simulink model "pjh_pid"  (R2020a)
settings: Solver=FixedStepAuto  StartTime=0.0  StopTime=inf  FixedStep=SAMPLE_TIME  RelTol=1e-3
undefined symbols (not defined in the file or in its folder): D_saturation, DiscIntNeverNeededParam, G_correct_gain, GEAR_RATIO, I_saturation, Kpid, Ktaud, MAX_QD, MAX_QDD, MAX_TAU, MJ_Test1_torque_mode, N, N_PLoop, N_VLoop, NUM_SEGMS, P_Kp, P_saturation, q_zero_offset, SAMPLE_TIME, theta_max, theta_min, v_des_saturation, V_Kd, V_Ki, V_Kp, v_threshold_I_stop
libraries: ighEthercatLib x38, simulink x7, simulink_extras x5, dspstat3 x3
(part 2 of 2)

== system pjh_pid/Enabled Subsystem1 ==
  In1 : Inport
  Enable : EnablePort
  Out1 : Outport
  wires:
  In1/1 -> Out1/1

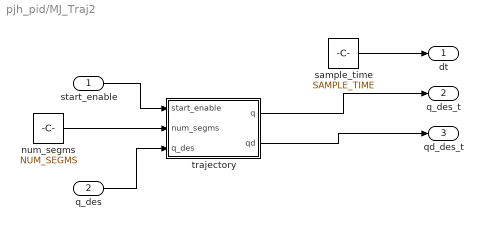
== system pjh_pid/MJ_Traj2 ==
  start_enable : Inport
  q_des : Inport  Port=2
  num_segms : Constant  Value=NUM_SEGMS
  sample_time : Constant  Value=SAMPLE_TIME
  trajectory : Subsystem
  dt : Outport
  q_des_t : Outport  Port=2
  qd_des_t : Outport  Port=3
  wires:
  sample_time/1 -> dt/1
  trajectory/1(q) -> q_des_t/1
  trajectory/2(qd) -> qd_des_t/1
  num_segms/1 -> trajectory/2(num_segms)
  start_enable/1 -> trajectory/1(start_enable)
  q_des/1 -> trajectory/3(q_des)

== system pjh_pid/Model Source ==

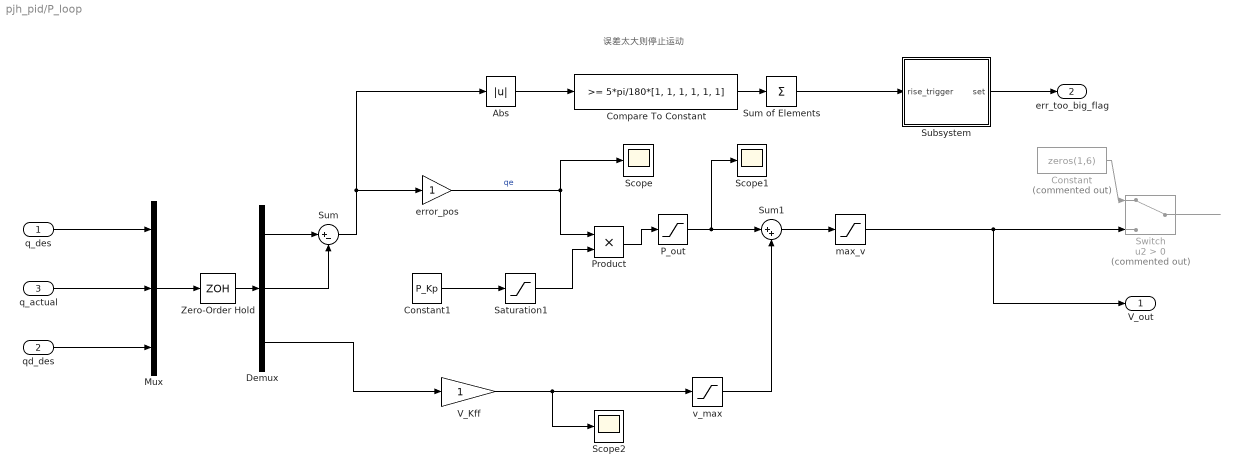
== system pjh_pid/P_loop ==
  note: 误差太大则停止运动
  q_des : Inport
  qd_des : Inport  Port=2
  q_actual : Inport  Port=3
  Abs : Abs
  Compare To Constant : simulink/Logic and Bit Operations/Compare To Constant  relop=>=  const=5*pi/180*[1, 1, 1, 1, 1, 1]  OutDataTypeStr=boolean
  Constant : Constant  Commented=on  Value=zeros(1,6)
  Constant1 : Constant  Value=P_Kp
  Demux : Demux  Outputs=[6 6 6]
  Mux : Mux  Inputs=3
  P_out : Saturate  UpperLimit=MAX_QD*0.8  LowerLimit=-MAX_QD*0.8
  Product : Product
  Saturation1 : Saturate  UpperLimit=50*ones(1,6)  LowerLimit=zeros(1,6)
  Scope : Scope
  Scope1 : Scope
  Scope2 : Scope
  Subsystem : Subsystem
  Sum : Sum  Inputs=|+-
  Sum of Elements : Sum  Inputs=+
  Sum1 : Sum  Inputs=|++
  Switch : Switch  Commented=on  Criteria=u2 > Threshold
  V_Kff : Gain
  Zero-Order Hold : ZeroOrderHold  SampleTime=SAMPLE_TIME*N_PLoop
  error_pos : Gain
  max_v : Saturate  UpperLimit=MAX_QD*4  LowerLimit=-MAX_QD*4
  v_max : Saturate  UpperLimit=MAX_QD*2  LowerLimit=-MAX_QD*2
  V_out : Outport
  err_too_big_flag : Outport  Port=2
  wires:
  Demux/1 -> Sum/1
  Product/1 -> P_out/1
  Demux/2 -> Sum/2
  Demux/3 -> V_Kff/1
  V_Kff/1 -> Scope2/1, v_max/1
  Sum1/1 -> max_v/1
  q_des/1 -> Mux/1
  q_actual/1 -> Mux/2
  qd_des/1 -> Mux/3
  Mux/1 -> Zero-Order Hold/1
  Zero-Order Hold/1 -> Demux/1
  max_v/1 -> V_out/1, Switch/3
  error_pos/1 -> Product/1, Scope/1  "qe"
  P_out/1 -> Sum1/1, Scope1/1
  Sum/1 -> error_pos/1, Abs/1
  v_max/1 -> Sum1/2
  Abs/1 -> Compare To Constant/1
  Switch/1 -> ?
  Constant/1 -> Switch/1
  Sum of Elements/1 -> Subsystem/1(rise_trigger)
  Compare To Constant/1 -> Sum of Elements/1
  Subsystem/1(set) -> err_too_big_flag/1
  Constant1/1 -> Saturation1/1
  Saturation1/1 -> Product/2

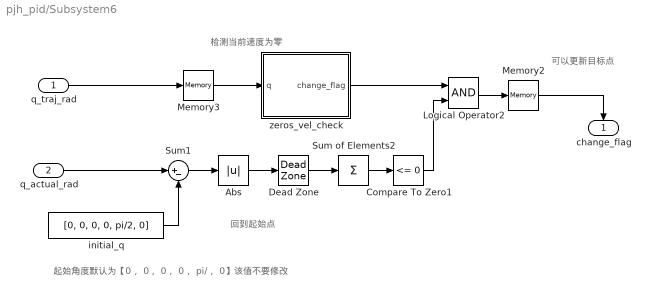
== system pjh_pid/Subsystem6 ==
  note: 起始角度默认为【0， 0， 0， 0， pi/， 0】该值不要修改
  note: 可以更新目标点
  note: 回到起始点
  note: 检测当前速度为零
  q_traj_rad : Inport
  q_actual_rad : Inport  Port=2
  Abs : Abs
  Compare To Zero1 : simulink/Logic and Bit Operations/Compare To Zero  relop=<=  OutDataTypeStr=boolean
  Dead Zone : DeadZone  LowerValue=zeros(1,6)  UpperValue=2*pi/180*[1, 1, 1, 1, 1, 1]  SaturateOnIntegerOverflow=on
  Logical Operator2 : Logic  AllPortsSameDT=off  OutDataTypeStr=boolean
  Memory2 : Memory  InitialCondition=1  InheritSampleTime=on
  Memory3 : Memory  InitialCondition=[0, 0, 0, 0, pi/2, 0]  InheritSampleTime=on
  Sum of Elements2 : Sum  Inputs=+
  Sum1 : Sum  Inputs=|+-
  initial_q : Constant  Value=[0, 0, 0, 0, pi/2, 0]
  zeros_vel_check : Subsystem
  change_flag : Outport
  wires:
  Logical Operator2/1 -> Memory2/1
  q_actual_rad/1 -> Sum1/1
  Abs/1 -> Dead Zone/1
  initial_q/1 -> Sum1/2
  Sum of Elements2/1 -> Compare To Zero1/1
  Compare To Zero1/1 -> Logical Operator2/2
  Sum1/1 -> Abs/1
  Dead Zone/1 -> Sum of Elements2/1
  zeros_vel_check/1(change_flag) -> Logical Operator2/1
  Memory3/1 -> zeros_vel_check/1(q)
  Memory2/1 -> change_flag/1
  q_traj_rad/1 -> Memory3/1

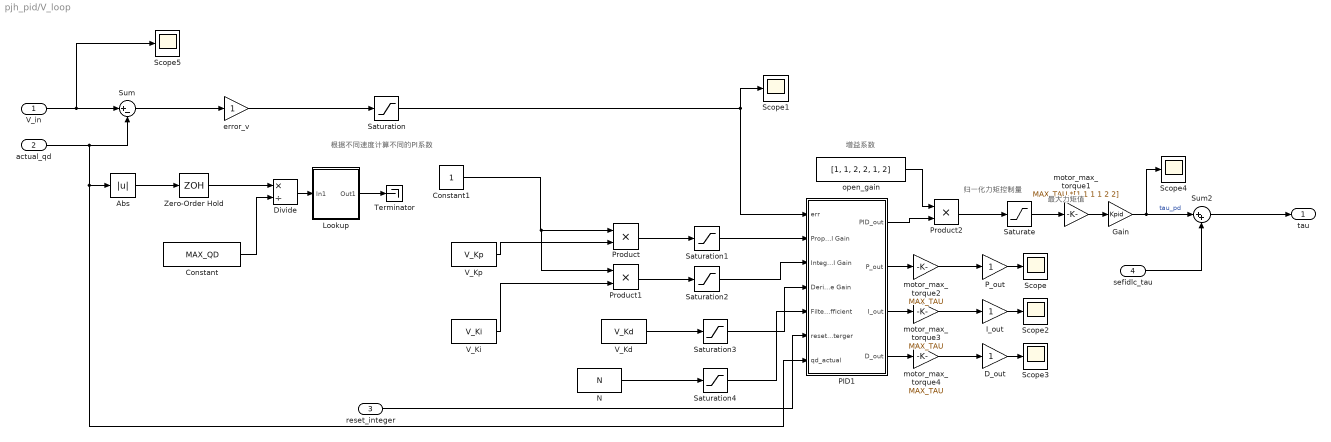
== system pjh_pid/V_loop ==
  note: 归一化力矩控制量
  note: 最大力矩值
  note: 增益系数
  note: 根据不同速度计算不同的PI系数
  V_in : Inport
  actual_qd : Inport  Port=2
  reset_integer : Inport  Port=3
  sefidlc_tau : Inport  Port=4
  " Lookup" : Subsystem
  Abs : Abs
  Constant : Constant  Value=MAX_QD
  Constant1 : Constant
  D_out : Gain
  Divide : Product  Inputs=*/
  Gain : Gain  Gain=Kpid
  I_out : Gain
  N : Constant  Value=N
  PID1 : Subsystem  AncestorBlock=simulink/Continuous/PID Controller  DialogController=pidpack.PIDConfig.pidDDGCreate
      settings: DeleteFcn=pidpack.PIDConfig.closeTuner(gcbh)  ModelCloseFcn=pidpack.PIDConfig.closeTuner(gcbh)  NameChangeFcn=pidpack.PIDConfig.updateTunerName(gcbh)
  P_out : Gain
  Product : Product
  Product1 : Product
  Product2 : Product
  Saturate : Saturate  UpperLimit=ones(1,6)  LowerLimit=-ones(1,6)
  Saturation : Saturate  UpperLimit=v_des_saturation*4  LowerLimit=-v_des_saturation*4
  Saturation1 : Saturate  UpperLimit=[10, 10, 10, 10, 10, 10]  LowerLimit=[0, 0, 0, 0, 0, 0]
  Saturation2 : Saturate  UpperLimit=200*[1, 1, 1, 1, 1, 1]  LowerLimit=[0, 0, 0, 0, 0, 0]
  Saturation3 : Saturate  UpperLimit=[10, 10, 10, 10, 10, 10]  LowerLimit=[0, 0, 0, 0, 0, 0]
  Saturation4 : Saturate  UpperLimit=[10, 10, 10, 10, 10, 10]  LowerLimit=[0, 0, 0, 0, 0, 0]
  Scope{,1..5} (6 alike) : Scope
  Sum : Sum  Inputs=|+-
  Sum2 : Sum  Inputs=|++
  Terminator : Terminator
  V_Kd : Constant  Value=V_Kd
  V_Ki : Constant  Value=V_Ki
  V_Kp : Constant  Value=V_Kp
  Zero-Order Hold : ZeroOrderHold  SampleTime=SAMPLE_TIME
  error_v : Gain
  motor_max_torque1 : Gain  Gain=MAX_TAU.*[1 1 1 1 2 2]
  motor_max_torque2 : Gain  Gain=MAX_TAU
  motor_max_torque3 : Gain  Gain=MAX_TAU
  motor_max_torque4 : Gain  Gain=MAX_TAU
  open_gain : Constant  Value=[1, 1, 2, 2, 1, 2]
  tau : Outport
  wires:
  V_in/1 -> Sum/1, Scope5/1
  actual_qd/1 -> PID1/7(qd_actual), Abs/1, Sum/2
  motor_max_torque1/1 -> Gain/1
  Sum/1 -> error_v/1
  error_v/1 -> Saturation/1
  Saturation/1 -> PID1/1(err), Scope1/1
  Saturation1/1 -> PID1/2(Proportional Gain)
  V_Kd/1 -> Saturation3/1
  N/1 -> Saturation4/1
  PID1/2(P_out) -> motor_max_torque2/1
  PID1/3(I_out) -> motor_max_torque3/1
  PID1/4(D_out) -> motor_max_torque4/1
  Product2/1 -> Saturate/1
  Product/1 -> Saturation1/1
  Saturation2/1 -> PID1/3(Integral Gain)
  Saturation3/1 -> PID1/4(Derivative Gain)
  Saturation4/1 -> PID1/5(Filter Coefficient)
  Abs/1 -> Zero-Order Hold/1
  Constant/1 -> Divide/2
  Divide/1 -> " Lookup"/1(In1)
  Zero-Order Hold/1 -> Divide/1
  motor_max_torque2/1 -> P_out/1
  Product1/1 -> Saturation2/1
  open_gain/1 -> Product2/1
  reset_integer/1 -> PID1/6(reset_interger)
  Sum2/1 -> tau/1
  V_Kp/1 -> Product/2
  V_Ki/1 -> Product1/2
  PID1/1(PID_out) -> Product2/2
  Saturate/1 -> motor_max_torque1/1
  Constant1/1 -> Product1/1, Product/1
  " Lookup"/1(Out1) -> Terminator/1
  P_out/1 -> Scope/1
  I_out/1 -> Scope2/1
  motor_max_torque3/1 -> I_out/1
  D_out/1 -> Scope3/1
  motor_max_torque4/1 -> D_out/1
  Gain/1 -> Scope4/1, Sum2/1  "tau_pd"
  sefidlc_tau/1 -> Sum2/2

== system pjh_pid/inc2rad ==
  inc : Inport
  Constant : Constant
  Divide : Product  Inputs=*/
  gear_ratio : Gain  Gain=GEAR_RATIO
  rad2inc : Gain  Gain=2^17/(2*pi)
  rad : Outport
  wires:
  gear_ratio/1 -> rad2inc/1
  rad2inc/1 -> Divide/2
  Constant/1 -> gear_ratio/1
  Divide/1 -> rad/1
  inc/1 -> Divide/1

== system pjh_pid/inc2rad1 ==
  inc : Inport
  Constant : Constant
  Divide : Product  Inputs=*/
  gear_ratio : Gain  Gain=GEAR_RATIO
  rad2inc : Gain  Gain=2^17/(2*pi)
  rad : Outport
  wires:
  inc/1 -> Divide/1
  Divide/1 -> rad/1
  Constant/1 -> gear_ratio/1
  rad2inc/1 -> Divide/2
  gear_ratio/1 -> rad2inc/1

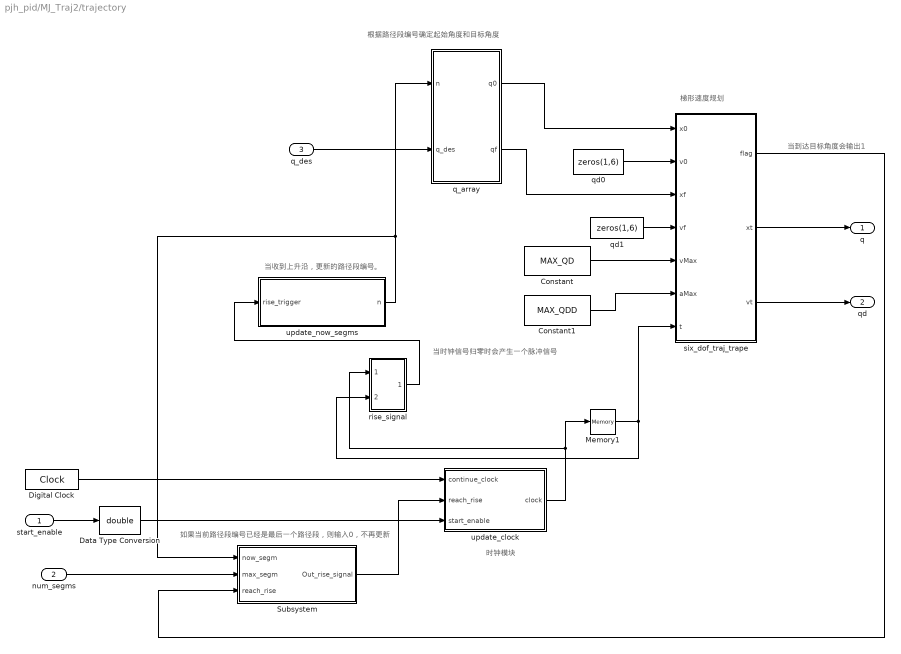
== system pjh_pid/MJ_Traj2/trajectory ==
  note: 如果当前路径段编号已经是最后一个路径段，则输入0，不再更新
  note: 当到达目标角度会输出1
  note: 根据路径段编号确定起始角度和目标角度
  note: 当收到上升沿，更新的路径段编号。
  note: 当时钟信号归零时会产生一个脉冲信号
  note: 时钟模块
  note: 梯形速度规划
  start_enable : Inport
  num_segms : Inport  Port=2
  q_des : Inport  Port=3
  Constant : Constant  Value=MAX_QD
  Constant1 : Constant  Value=MAX_QDD
  Data Type Conversion : DataTypeConversion  OutDataTypeStr=double
  Digital Clock : DigitalClock  SampleTime=SAMPLE_TIME
  Memory1 : Memory
  Subsystem : Subsystem
  q_array : MATLAB Function  TreatAsAtomicUnit=on  SystemSampleTime=SAMPLE_TIME
  qd0 : Constant  Value=zeros(1,6)
  qd1 : Constant  Value=zeros(1,6)
  rise_signal : Subsystem
  six_dof_traj_trape : MATLAB Function  TreatAsAtomicUnit=on
  update_clock : Subsystem
  update_now_segms : Subsystem
  q : Outport
  qd : Outport  Port=2
  wires:
  q_array/2(qf) -> six_dof_traj_trape/3(xf)
  Digital Clock/1 -> update_clock/1(continue_clock)
  Memory1/1 -> six_dof_traj_trape/7(t), rise_signal/2(In2)
  q_array/1(q0) -> six_dof_traj_trape/1(x0)
  rise_signal/1(Out1) -> update_now_segms/1(rise_trigger)
  update_clock/1(clock) -> rise_signal/1(In1), Memory1/1
  Subsystem/1(Out_rise_signal) -> update_clock/2(reach_rise)
  num_segms/1 -> Subsystem/2(max_segm)
  update_now_segms/1(n) -> q_array/1(n), Subsystem/1(now_segm)
  six_dof_traj_trape/2(xt) -> q/1
  six_dof_traj_trape/3(vt) -> qd/1
  qd0/1 -> six_dof_traj_trape/2(v0)
  qd1/1 -> six_dof_traj_trape/4(vf)
  six_dof_traj_trape/1(flag) -> Subsystem/3(reach_rise)
  Data Type Conversion/1 -> update_clock/3(start_enable)
  start_enable/1 -> Data Type Conversion/1
  q_des/1 -> q_array/2(q_des)
  Constant/1 -> six_dof_traj_trape/5(vMax)
  Constant1/1 -> six_dof_traj_trape/6(aMax)

== system pjh_pid/P_loop/Subsystem ==
  rise_trigger : Inport
  Constant1 : Constant
  Memory2 : Memory  InheritSampleTime=on
  Triggered Subsystem1 : Subsystem  TreatAsAtomicUnit=on
  set : Outport
  wires:
  rise_trigger/1 -> Triggered Subsystem1/Trigger
  Triggered Subsystem1/1(Out1) -> Memory2/1
  Constant1/1 -> Triggered Subsystem1/1(In1)
  Memory2/1 -> set/1

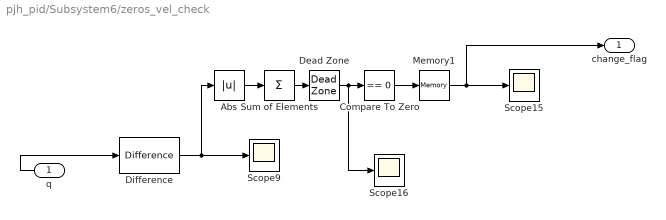
== system pjh_pid/Subsystem6/zeros_vel_check ==
  q : Inport
  Abs : Abs
  Compare To Zero : simulink/Logic and Bit Operations/Compare To Zero  relop===  OutDataTypeStr=boolean
  Dead Zone : DeadZone  LowerValue=0  UpperValue=0.0001  SaturateOnIntegerOverflow=on
  Difference : simulink/Discrete/Difference  ICPrevInput=zeros(1,6)  OutMin=[]  OutMax=[]  OutDataType=fixdt(1, 16)  OutScaling=2^-10  DoSatur=off
  Memory1 : Memory  InitialCondition=1  InheritSampleTime=on
  Scope15 : Scope
  Scope16 : Scope
  Scope9 : Scope
  Sum of Elements : Sum  Inputs=+
  change_flag : Outport
  wires:
  q/1 -> Difference/1
  Abs/1 -> Sum of Elements/1
  Dead Zone/1 -> Compare To Zero/1, Scope16/1
  Memory1/1 -> change_flag/1, Scope15/1
  Difference/1 -> Scope9/1, Abs/1
  Compare To Zero/1 -> Memory1/1
  Sum of Elements/1 -> Dead Zone/1

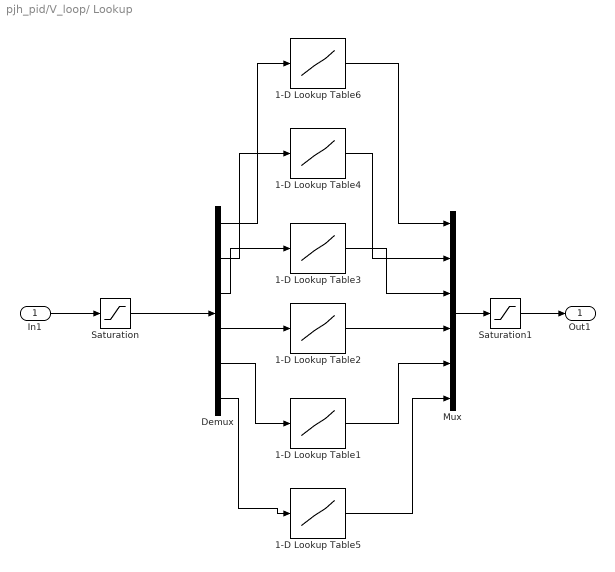
== system pjh_pid/V_loop/ Lookup ==
  In1 : Inport
  1-D Lookup Table{1..4,6} (5 alike) : Lookup_n-D  NumberOfTableDimensions=1  BreakpointsForDimension1=[0, 0.1,0.2, 0.3, 0.4, 1 ]  Table=[1, 1, 0.8, 0.6, 0.5, 0.5]  InternalRulePriority=Speed  RndMeth=Simplest  InputSameDT=on
  1-D Lookup Table5 : Lookup_n-D  NumberOfTableDimensions=1  BreakpointsForDimension1=[0, 0.1,0.2, 0.3, 0.4, 1 ]  Table=[1, 1, 1, 1, 1, 1]  InternalRulePriority=Speed  RndMeth=Simplest  InputSameDT=on
  Demux : Demux  Outputs=6
  Mux : Mux  Inputs=6
  Saturation : Saturate  UpperLimit=ones(1,6)  LowerLimit=zeros(1,6)
  Saturation1 : Saturate  UpperLimit=5*ones(1,6)  LowerLimit=zeros(1,6)
  Out1 : Outport
  wires:
  1-D Lookup Table6/1 -> Mux/1
  Demux/1 -> 1-D Lookup Table6/1
  In1/1 -> Saturation/1
  Demux/2 -> 1-D Lookup Table4/1
  Demux/3 -> 1-D Lookup Table3/1
  Demux/4 -> 1-D Lookup Table2/1
  Demux/5 -> 1-D Lookup Table1/1
  Demux/6 -> 1-D Lookup Table5/1
  Saturation/1 -> Demux/1
  1-D Lookup Table4/1 -> Mux/2
  1-D Lookup Table3/1 -> Mux/3
  1-D Lookup Table2/1 -> Mux/4
  1-D Lookup Table1/1 -> Mux/5
  1-D Lookup Table5/1 -> Mux/6
  Saturation1/1 -> Out1/1
  Mux/1 -> Saturation1/1

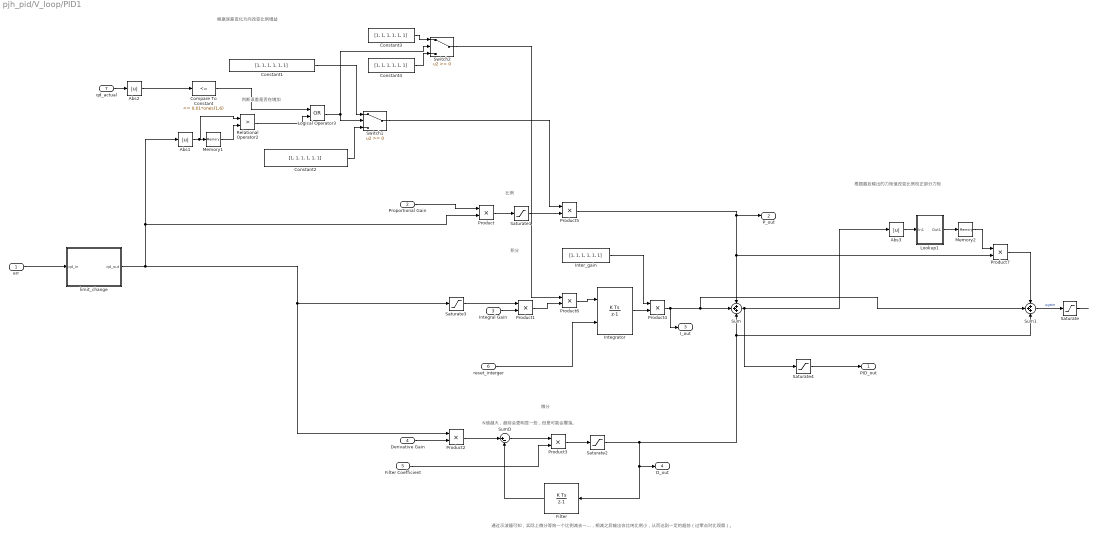
== system pjh_pid/V_loop/PID1 ==
  note: 根据最后输出的力矩值改变比例校正部分力矩
  note: 根据误差变化方向改变比例增益
  note: 判断误差是否在增加
  note: 通过示波器可知，实际上微分等效一个比例减去一个积分。比例持续正输出，则积分反馈不断增加，相减之后输出会比纯比例小，从而达到一定的超前（过零点对比观察）。
  note: 微分
  note: 积分
  note: 比例
  note: N值越大，超前会更明显一些，但是可能会震荡。
  err : Inport
  Proportional Gain : Inport  Port=2
  Integral Gain : Inport  Port=3
  Derivative Gain : Inport  Port=4
  Filter Coefficient : Inport  Port=5
  reset_interger : Inport  Port=6
  qd_actual : Inport  Port=7
  " Lookup1" : Subsystem
  Abs1 : Abs
  Abs2 : Abs
  Abs3 : Abs
  Compare To Constant : simulink/Logic and Bit Operations/Compare To Constant  relop=<=  const=0.01*ones(1,6)  OutDataTypeStr=boolean
  Constant{1..4} (4 alike) : Constant  Value=[1, 1, 1, 1, 1, 1]
  Filter : DiscreteIntegrator  DisableCoverage=on  SampleTime=-1  ICPrevOutput=DiscIntNeverNeededParam  ICPrevScaledInput=DiscIntNeverNeededParam
  Integrator : DiscreteIntegrator  ExternalReset=level  InitialCondition=zeros(1,6)  SampleTime=-1  LimitOutput=on  UpperSaturationLimit=I_saturation  LowerSaturationLimit=-I_saturation  ICPrevOutput=DiscIntNeverNeededParam  ICPrevScaledInput=DiscIntNeverNeededParam
  Inter_gain : Constant  Value=[1, 1, 1, 1, 1, 1]
  Logical Operator3 : Logic  Operator=OR  AllPortsSameDT=off  OutDataTypeStr=boolean
  Memory1 : Memory  InitialCondition=zeros(1,6)  InheritSampleTime=on
  Memory2 : Memory  InitialCondition=ones(1,6)  InheritSampleTime=on
  Product{,1..7} (8 alike) : Product
  Relational Operator2 : RelationalOperator  Operator=>  OutDataTypeStr=boolean  RndMeth=Simplest
  Saturate : Saturate  UpperLimit=ones(1,6)  LowerLimit=-ones(1,6)
  Saturate1 : Saturate  UpperLimit=P_saturation  LowerLimit=-P_saturation
  Saturate2 : Saturate  UpperLimit=D_saturation  LowerLimit=-D_saturation
  Saturate3 : Saturate  UpperLimit=v_threshold_I_stop  LowerLimit=-v_threshold_I_stop
  Saturate4 : Saturate  UpperLimit=ones(1,6)  LowerLimit=-ones(1,6)
  Sum : Sum  Inputs=+++
  Sum1 : Sum  Inputs=+++
  SumD : Sum  DisableCoverage=on  Inputs=|+-
  Switch1 : Switch
  Switch2 : Switch
  limit_change : Subsystem
  PID_out : Outport  InitialOutput=0
  P_out : Outport  Port=2  InitialOutput=0
  I_out : Outport  Port=3  InitialOutput=0
  D_out : Outport  Port=4  InitialOutput=0
  wires:
  Product4/1 -> I_out/1, Sum/2, Sum1/2
  Product2/1 -> SumD/1
  SumD/1 -> Product3/1
  Saturate2/1 -> Filter/1, D_out/1, Sum1/3, Sum/3
  Filter/1 -> SumD/2
  Saturate/1 -> ?
  Product/1 -> Saturate1/1
  Product3/1 -> Saturate2/1
  Proportional Gain/1 -> Product/1
  Integral Gain/1 -> Product1/2
  Derivative Gain/1 -> Product2/2
  Filter Coefficient/1 -> Product3/2
  limit_change/1(qd_out) -> Product2/1, Saturate3/1, Abs1/1, Product/2
  Integrator/1 -> Product4/2
  Inter_gain/1 -> Product4/1
  reset_interger/1 -> Integrator/2
  Product1/1 -> Product6/2
  Abs1/1 -> Relational Operator2/1, Memory1/1
  Memory1/1 -> Relational Operator2/2
  Constant1/1 -> Switch1/1
  Logical Operator3/1 -> Switch1/2, Switch2/2
  Constant2/1 -> Switch1/3
  Saturate1/1 -> Product5/2
  Switch1/1 -> Product5/1
  qd_actual/1 -> Abs2/1
  Abs2/1 -> Compare To Constant/1
  Relational Operator2/1 -> Logical Operator3/2
  Compare To Constant/1 -> Logical Operator3/1
  Product6/1 -> Integrator/1
  Constant3/1 -> Switch2/1
  Constant4/1 -> Switch2/3
  Switch2/1 -> Product6/1
  Sum/1 -> Saturate4/1, Abs3/1
  Abs3/1 -> " Lookup1"/1(In1)
  " Lookup1"/1(Out1) -> Memory2/1
  Memory2/1 -> Product7/1
  Product5/1 -> Sum/1, Product7/2, P_out/1
  Product7/1 -> Sum1/1
  Saturate3/1 -> Product1/1
  Saturate4/1 -> PID_out/1
  err/1 -> limit_change/1(qd_in)
  Sum1/1 -> Saturate/1  "ugain"

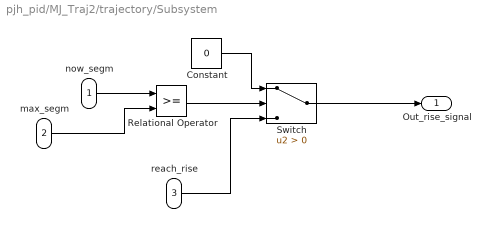
== system pjh_pid/MJ_Traj2/trajectory/Subsystem ==
  now_segm : Inport
  max_segm : Inport  Port=2
  reach_rise : Inport  Port=3
  Constant : Constant  Value=0
  Relational Operator : RelationalOperator  OutDataTypeStr=boolean  RndMeth=Simplest
  Switch : Switch  Criteria=u2 > Threshold
  Out_rise_signal : Outport
  wires:
  now_segm/1 -> Relational Operator/1
  reach_rise/1 -> Switch/3
  max_segm/1 -> Relational Operator/2
  Relational Operator/1 -> Switch/2
  Switch/1 -> Out_rise_signal/1
  Constant/1 -> Switch/1

== system pjh_pid/MJ_Traj2/trajectory/rise_signal ==
  In1 : Inport
  In2 : Inport  Port=2
  Delay : Delay  DelayLength=1
  Relational Operator : RelationalOperator  Operator=<  OutDataTypeStr=boolean  RndMeth=Simplest
  Out1 : Outport
  wires:
  In2/1 -> Delay/1
  In1/1 -> Relational Operator/1
  Delay/1 -> Relational Operator/2
  Relational Operator/1 -> Out1/1

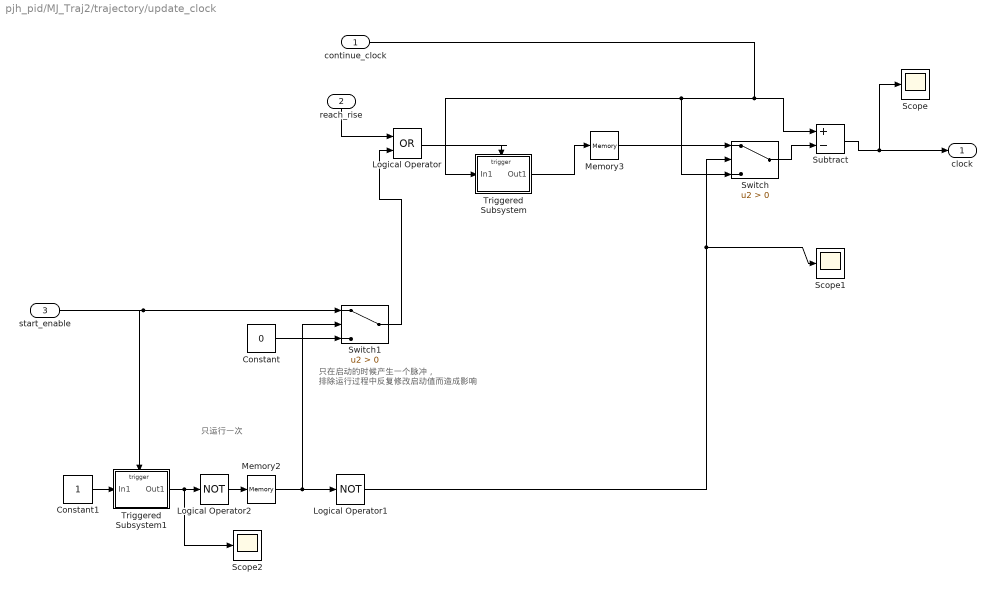
== system pjh_pid/MJ_Traj2/trajectory/update_clock ==
  note: 只在启动的时候产生一个脉冲，
      | 排除运行过程中反复修改启动值而造成影响
  note: 只运行一次
  continue_clock : Inport
  reach_rise : Inport  Port=2
  start_enable : Inport  Port=3
  Constant : Constant  Value=0
  Constant1 : Constant
  Logical Operator : Logic  Operator=OR  AllPortsSameDT=off  OutDataTypeStr=boolean
  Logical Operator1 : Logic  Operator=NOT  AllPortsSameDT=off  OutDataTypeStr=boolean
  Logical Operator2 : Logic  Operator=NOT  AllPortsSameDT=off  OutDataTypeStr=boolean
  Memory2 : Memory  InitialCondition=1
  Memory3 : Memory
  Scope : Scope
  Scope1 : Scope
  Scope2 : Scope
  Subtract : Sum  Inputs=+-
  Switch : Switch  Criteria=u2 > Threshold
  Switch1 : Switch  Criteria=u2 > Threshold
  Triggered Subsystem : Subsystem  TreatAsAtomicUnit=on
  Triggered Subsystem1 : Subsystem  TreatAsAtomicUnit=on
  clock : Outport
  wires:
  Memory3/1 -> Switch/1
  continue_clock/1 -> Switch/3, Triggered Subsystem/1(In1), Subtract/1
  reach_rise/1 -> Logical Operator/1
  Subtract/1 -> Scope/1, clock/1
  Triggered Subsystem/1(Out1) -> Memory3/1
  Switch/1 -> Subtract/2
  Logical Operator/1 -> Triggered Subsystem/Trigger
  start_enable/1 -> Switch1/1, Triggered Subsystem1/Trigger
  Switch1/1 -> Logical Operator/2
  Triggered Subsystem1/1(Out1) -> Logical Operator2/1, Scope2/1
  Memory2/1 -> Switch1/2, Logical Operator1/1
  Constant/1 -> Switch1/3
  Logical Operator1/1 -> Scope1/1, Switch/2
  Constant1/1 -> Triggered Subsystem1/1(In1)
  Logical Operator2/1 -> Memory2/1

== system pjh_pid/MJ_Traj2/trajectory/update_now_segms ==
  rise_trigger : Inport
  Memory2 : Memory
  Subsystem3 : Subsystem
  Switch3 : Switch  Criteria=u2 > Threshold  Threshold=1
  inital_segm_const : Constant
  n : Outport
  wires:
  Switch3/1 -> n/1
  Memory2/1 -> Switch3/2, Switch3/1
  Subsystem3/1(n) -> Memory2/1
  inital_segm_const/1 -> Switch3/3
  rise_trigger/1 -> Subsystem3/Trigger

== system pjh_pid/P_loop/Subsystem/Triggered Subsystem1 ==
  In1 : Inport
  Trigger : TriggerPort  VariantControl=Variant
  Out1 : Outport
  wires:
  In1/1 -> Out1/1

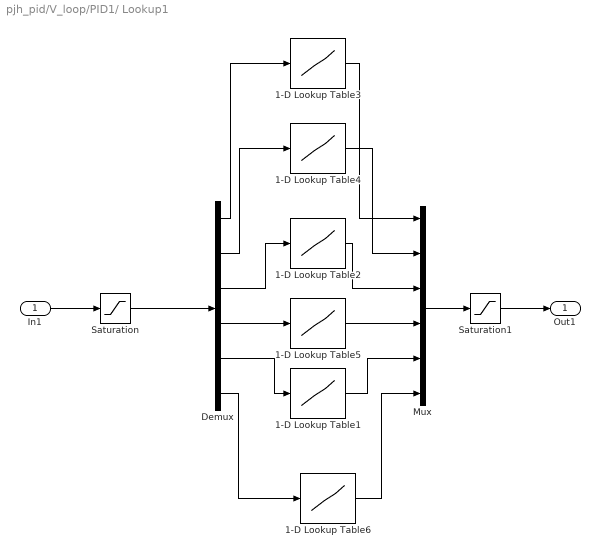
== system pjh_pid/V_loop/PID1/ Lookup1 ==
  In1 : Inport
  1-D Lookup Table1 : Lookup_n-D  NumberOfTableDimensions=1  BreakpointsForDimension1="[0, 0.03, 0.12,  1 ]"  Table="[1, 1,  0.5,  0.5]"  InternalRulePriority=Speed  RndMeth=Simplest  InputSameDT=on
  1-D Lookup Table2 : Lookup_n-D  NumberOfTableDimensions=1  BreakpointsForDimension1="[0, 0.03, 0.12,  1 ]"  Table="[1, 1,  1,  1]"  InternalRulePriority=Speed  RndMeth=Simplest  InputSameDT=on
  1-D Lookup Table3 : Lookup_n-D  NumberOfTableDimensions=1  BreakpointsForDimension1="[0, 0.03, 0.12,  1 ]"  Table="[1, 1,  1,  1]"  InternalRulePriority=Speed  RndMeth=Simplest  InputSameDT=on
  1-D Lookup Table4 : Lookup_n-D  NumberOfTableDimensions=1  BreakpointsForDimension1="[0, 0.02, 0.08,  1 ]"  Table="[1, 1,  0.5,  0.4]"  InternalRulePriority=Speed  RndMeth=Simplest  InputSameDT=on
  1-D Lookup Table5 : Lookup_n-D  NumberOfTableDimensions=1  BreakpointsForDimension1="[0, 0.03, 0.12,  1 ]"  Table="[1, 1,  1,  1]"  InternalRulePriority=Speed  RndMeth=Simplest  InputSameDT=on
  1-D Lookup Table6 : Lookup_n-D  NumberOfTableDimensions=1  BreakpointsForDimension1="[0, 0.03, 0.12,  1 ]"  Table="[1, 1,  0.4,  0.4]"  InternalRulePriority=Speed  RndMeth=Simplest  InputSameDT=on
  Demux : Demux  Outputs=6
  Mux : Mux  Inputs=6
  Saturation : Saturate  UpperLimit=ones(1,6)  LowerLimit=zeros(1,6)
  Saturation1 : Saturate  UpperLimit=ones(1,6)  LowerLimit=zeros(1,6)
  Out1 : Outport
  wires:
  1-D Lookup Table3/1 -> Mux/1
  Demux/1 -> 1-D Lookup Table3/1
  In1/1 -> Saturation/1
  Demux/2 -> 1-D Lookup Table4/1
  Demux/3 -> 1-D Lookup Table2/1
  Demux/4 -> 1-D Lookup Table5/1
  Demux/5 -> 1-D Lookup Table1/1
  Demux/6 -> 1-D Lookup Table6/1
  Saturation/1 -> Demux/1
  1-D Lookup Table4/1 -> Mux/2
  1-D Lookup Table2/1 -> Mux/3
  1-D Lookup Table5/1 -> Mux/4
  1-D Lookup Table1/1 -> Mux/5
  1-D Lookup Table6/1 -> Mux/6
  Saturation1/1 -> Out1/1
  Mux/1 -> Saturation1/1

== system pjh_pid/V_loop/PID1/limit_change ==
  qd_in : Inport
  Memory : Memory  InheritSampleTime=on
  Saturation1 : Saturate  UpperLimit=MAX_QDD*SAMPLE_TIME*N_VLoop*150  LowerLimit=-MAX_QDD*SAMPLE_TIME*N_VLoop*150
  Sum3 : Sum  Inputs=|+-
  Sum4 : Sum  Inputs=|++
  qd_out : Outport
  wires:
  Sum3/1 -> Saturation1/1
  Sum4/1 -> Memory/1
  Memory/1 -> qd_out/1, Sum4/2, Sum3/2
  Saturation1/1 -> Sum4/1
  qd_in/1 -> Sum3/1

== system pjh_pid/MJ_Traj2/trajectory/update_clock/Triggered Subsystem ==
  In1 : Inport
  Trigger : TriggerPort  VariantControl=Variant
  Out1 : Outport
  wires:
  In1/1 -> Out1/1

== system pjh_pid/MJ_Traj2/trajectory/update_clock/Triggered Subsystem1 ==
  In1 : Inport
  Trigger : TriggerPort  VariantControl=Variant
  Out1 : Outport
  wires:
  In1/1 -> Out1/1

== system pjh_pid/MJ_Traj2/trajectory/update_now_segms/Subsystem3 ==
  Trigger : TriggerPort  VariantControl=Variant
  Add : Sum
  Memory2 : Memory  InitialCondition=2  InheritSampleTime=on
  plus_one : Constant
  n : Outport
  wires:
  Memory2/1 -> Add/1, n/1
  Add/1 -> Memory2/1
  plus_one/1 -> Add/2

== matlab function pjh_pid/MJ_frict_compen1 ==
  data: qd input size=[1 6]; fric_new output size=[1 6]
function fric_new  = fcn(qd)
     X=[5.9994    5.9994    0.0000    0.2252;
      -31.2146   37.6169    0.0089    0.6627;
      6.5893    6.5893         0    0.3293;
      15.1083    2.9149    0.4581    0.1456;
      5.9167    5.9167         0    0.1172;
      8.9388    2.1631    0.5005    0.1224];%提前辨识出来，2023.9.8
 fric_new=zeros(1,6)  ;
for i=1:6
    y=X(i,:);
fric_new(i)=fun(y,57.29*abs(qd(i)))*sign(qd(i));
end

end

== matlab function pjh_pid/MATLAB Function1 ==
  data: t input; q output; qd output; qdd output
function [q,qd,qdd] = fcn(t)
% persistent a;persistent f;persistent I;persistent b;
% t(t>200)=200;
% if isempty(a)
% %     rng('shuffle');
%     a=randn(10,6);
%     f=randn(10,6)*0.2*pi+0.1*pi;
%     b=randn(10,6)*2*pi;
%     I=10;
% end
% if t>I
%     a=randn(10,6);
%     f=randn(10,6)*0.2*pi+0.1*pi;
%     b=randn(10,6)*2*pi;
%     I=I+10;
% end
% B=[60 40 50 60 60 90]*pi/180;
% mean(a)
% q=[B.*sum(a.*sin(f*t+b))/5]'+[0 -20 -20 0 0 0]'*pi/180;
% qd=[B.*sum(a.*f.*cos(f*t+b))/5]';
% qdd=[B.*sum(-a.*f.*f.*sin(f*t+b))/5]';

% t(t>40)=40;
fq=0.2*pi;
B=[30 20 -30 30 -30 -30]*pi/180;
q0=[10 -20 -20 10 15 0]'*pi/180;
q=[B.*sin(fq*t)]'+q0;
qd=[B.*fq.*cos(fq*t)]';
qdd=[-B.*fq.*fq.*sin(fq*t)]';
% q(4:6)=0;qd(4:6)=0;qdd(4:6)=0;
if t==40
    qd=zeros(6,1);qdd=zeros(6,1);
end
if t==0
    q=[0; 0 ;0 ;0; 0; 0];qd=zeros(6,1);qdd=zeros(6,1);
end
end

== matlab function pjh_pid/MATLAB Function ==
  data: q input; taud output; qd input; t input
function taud  = dis(q,qd,t)

taud=1*[20; 20 ;20 ;10 ;5 ;2]*sin(0.3*pi*t)+[10; 10; 10; 5; 5; 1].*sin(q)+[1; 1; 1; 0.5; 0.5; 0.5].*qd;

== matlab function pjh_pid/MATLAB Function4 ==
  settings: updateMethod=DISCRETE
  data: q output; q input; qd output; qdd output
function [q,qd,qdd] = fcn(q)
persistent x0;persistent x1;persistent x2;
if isempty(x0)
    x0=q;
    x1=0*q;
    x2=0*q;
end
dt=0.0005;
k0=x1-100*abs(x0-q).^(2/3).*sign(x0-q);
k1=x2-20*abs(x1-k0).^(1/2).*sign(x1-k0);
% k2=m3*sign(k1-x2);
k2=10*(k1-x2);
x0=x0+k0*dt;
x1=x1+k1*dt;
x2=x2+k2*dt;
q=x0;
qd=x1;
qdd=x2;

== matlab function pjh_pid/MJ_G_compen ==
  data: q_actual input size=[1 6]; G_tau output size=[1 6]
function G_tau = MJ_G_vector_pack(q_actual)
    G_tau = MJ_G_vector( q_actual );
end

== matlab function pjh_pid/MJ_M_matic ==
  data: q input size=[1 6]; M output size=[6 6]
function M = MJ_M_matic_pack(q)
    [ M ] = MJ_M_matric( q );
end

== matlab function pjh_pid/MJ_TAU ==
  data: q input size=[1 6]; ALL_tau output size=[1 6]; qd input size=[1 6]; qdd input size=[1 6]; f_ext input size=[1 3]; n_ext input size=[1 3]; grav input size=[1 3]
function ALL_tau = MJ_rne_pack( q, qd, qdd, f_ext, n_ext, grav)
[ ALL_tau, wbase ] = MJ_rne( q, qd, qdd, f_ext, n_ext, grav);
end

== matlab function pjh_pid/MJ_Traj2/trajectory/q_array ==
  data: n input; q0 output size=[1 6]; qf output size=[1 6]; q_des input size=[1 6]
function [q0, qf] = fcn(n, q_des)
%%
%测试重力项
    q_array = [0.0,     0.0,	0.0,	0.0,	pi/2,	0.0;       %起始角度  默认为【0.0,     0.0,	0.0,	0.0,	pi/2,	0.0】
               0.0,     0.0,	0.0,	0.0,	0.0,	0.0];       %目标角度    
    q_array(2, :) = q_des;
%%
    if n < 1
        n =1;
    end           
    len = size(q_array, 1);
    k = mod(n, 2*(len-1));
    if 1<= k && k <= (len-1)
        q0 = q_array(k, :);
        qf = q_array(k+1, :);
    elseif (len-1) <k && k <= (2*(len-1) -1)
        q0 = q_array(2*len - k, :);
        qf = q_array(2*len - k - 1, :);
    else 
        q0 = q_array(2, :);
        qf = q_array(1, :);
    end
end

== matlab function pjh_pid/MJ_Traj2/trajectory/six_dof_traj_trape ==
  data: x0 input size=[1 6]; flag output; v0 input size=[1 6]; xf input size=[1 6]; vf input size=[1 6]; vMax input size=[1 6]; aMax input size=[1 6]; t input; xt output size=[1 6]; vt output size=[1 6]
function [flag, xt, vt] = traj_trape( x0,v0,xf,vf,vMax,aMax, t )
    %如果误差很小表示已经到达目标点。
    equal_1 = sum(abs(x0 - xf)) < 0.0001;
    equal_2 = sum(abs(v0 - zeros(1,6))) < 0.0001;
    equal_3 = sum(abs(vf - zeros(1,6))) < 0.0001;
    if equal_1 && equal_2 && equal_3
        flag = 1;
        xt = xf;
        vt = zeros(1,6);
        return;
    end
    [flag, xt, vt,test ] = six_dof_traj( x0,v0,xf,vf,vMax,aMax, t );
end

function [flag, xt, vt,test ] = six_dof_traj( x0,v0,xf,vf,vMax,aMax, t )
%SIX_DOF_TRAJ 
%   此处显示详细说明
%
len =length(x0);

bangBangBool = zeros(1,len);
a0 = zeros(1,len);
b0 = zeros(1,len);
c0 = zeros(1,len);
a1 = zeros(1,len);
b1 = zeros(1,len);
a2 = zeros(1,len);
b2 = zeros(1,len);
c2 = zeros(1,len);
t1 = zeros(1,len);
t2 = zeros(1,len);
tf = zeros(1,len);
reach_flag = zeros(1,len);

v_use = vMax;
a_use = aMax;

t_max = 0;
plotBool = 0;
%%
%computer trajectory
for n = 1:2
    for i = 1:len
        [bangBangBool(i),a0(i),b0(i),c0(i),a1(i),b1(i),a2(i),b2(i),c2(i),t1(i),t2(i),tf(i)] = getMinTimeTrajCoeffs(x0(i),v0(i),xf(i),vf(i),v_use(i),a_use(i));
        if tf(i) > t_max
            t_max = tf(i);
        end
    end
    %第二次就直接跳出了
    if n==2
        break;
    end
    
    v_use = abs(xf - x0)/t_max;
    for i = 1:len
        if v_use(i) < abs(v0(i))
            v_use(i) = abs(v0(i));
        end
    end
    a_use = (aMax./vMax) .* v_use;
end
%%
%ouput_value
xt = ones(1,len);
vt = ones(1,len);

for i = 1:len
    if bangBangBool(i) == 0     %have line
        if t<t1(i)
         	xt(i) = a0(i) + b0(i)*t + c0(i)*t^2;
            vt(i) = b0(i) + 2*c0(i)*t;
        elseif  t <=t2(i)
            xt(i) = a1(i) + b1(i)*t;
            vt(i) = b1(i);
        elseif t <= tf(i)
            xt(i) = a2(i) + b2(i)*t + c2(i)*t^2;
            vt(i) = b2(i) + 2*c2(i)*t;
        else
            xt(i) = xf(i);
            vt(i) = vf(i);
            reach_flag(i) = 1;
        end
        test = 100;
    else                        %have not line
        if t<=t2(i)
         	xt(i) = a0(i) + b0(i)*t + c0(i)*t^2;
            vt(i) = b0(i) + 2*c0(i)*t;
        elseif t <= tf(i)
            xt(i) = a2(i) + b2(i)*t + c2(i)*t^2;
            vt(i) = b2(i) + 2*c2(i)*t;
        else
            xt(i) = xf(i);
            vt(i) = vf(i);
            reach_flag(i) = 1;
        end
        test = 200;
    end 
%  test = tf(1);  

end

%%
% judge whether reach target
for i = 1:len
    if reach_flag(i) ~= 1
        flag = 0;
        break;
    end
    flag = 1;
end
end

%
% single dof traj
% 
function [bangBangBool,a0,b0,c0,a1,b1,a2,b2,c2,t1,t2,tf] = getMinTimeTrajCoeffs(x0,v0,xf,vf,vMax,aMax)
% Calculate the coefficients that define the three segments of an LSPB
% trajectory between state [x0,v0] and [xf,vf]. This code assumes maximum speed and
% acceleration are independent of direction.  Note that the acceleration is
% either -aMax, 0, or aMax at all times.  The resulting LSPB trajectory is
% the fastest trajectory possible that meets these velocity and
% acceleration constraints.

% Input:
%       x0: Initial position
%       v0: Initial velocity
%       xf: Final position
%       vf: Final velocity
%       vMax: Maximum allowed speed (either direction)
%       aMax: Maximum allowed acceleration (either direction)
%       plotBool: Set to 1 to generate a simple plot of the LSPB

% Output:
%       bangBangBool: 0 indicates that the trajectory contains a linear
%           portion, meaning all coefficients and output t's are required.
%           1 indicates that a linear portion is not required, thus the a1,
%           b1, and t1 output values will all be zero and can be ignored.
%       a0,b0,c0: Define first segment of LSPB (parabolic).  
%           For 0<=t<=t1, x = a0 + b0*t + c0*t^2
%       a1,b1: Define second segment of LSPB (linear).  
%           For t1<=t<=t2, x = a1 + b1*t 
%       a2,b2,c2: Define third segment of LSPB (parabolic).  
%           For t2<=t<=tf, x = a2 + b2*t + c2*t^2
%       t1,t2,tf: Times at which the above equations hold.

% Eric Young, 2018

%Check for errors
if(0>vMax)
    error('vMax must be positive')
end
if(0>aMax)
    error('aMax must be positive')
end
if(v0>vMax)
    error('Initial velocity is greater than vMax')
end
if(v0<-vMax)
    error('Initial velocity is less than -vMax')
end
if(vf>vMax)
    error('Final velocity is greater than vMax')
end
if(vf<-vMax)
    error('Final velocity is less than -vMax')
end


% First calculate maximum distance possible without linear segment
xfMaxBangBang = x0 + (vMax^2 - v0^2)/(2*aMax) + (vMax^2 - vf^2)/(2*aMax);

% Distance with only one parabolic blend (later used to determine if the
% first parabolic segment should have positive or negative
% acceleration)
if(vf>=v0)
    xfBang = x0 + (vf^2 - v0^2)/(2*aMax);
else
    xfBang = x0 + (v0^2 - vf^2)/(2*aMax);%xfBang = x0 + (vf^2 - v0^2)/(2*-aMax);
end

% Minimum distance possible without linear segment
xfMinBangBang = x0 + (vMax^2 - v0^2)/(2*-aMax) + (vMax^2 - vf^2)/(2*-aMax);

% Determine acceleration for first segment.  n = 1: begin with positive
% acceleration
if(xf>xfMaxBangBang)
    n = 1;
    bangBangBool = 0;
elseif(xf<xfMinBangBang)
    n = -1;
    bangBangBool = 0;
else
    bangBangBool = 1;
    if(xf>=xfBang)
        n = 1;
    else
        n = -1;
    end
end

% True for all cases
a0 = x0;
b0 = v0;
c0 = n*aMax/2;
c2 = -n*aMax/2;

%If no linear segment is needed (just a bang-bang trajectory)
if(bangBangBool)
    % Ignore linear portion
    t1 = 0;
    a1 = 0;
    b1 = 0;
    
    m = sqrt(2*c0*(xf-x0)+v0^2/2+vf^2/2);
    t2 = (-b0+m)/(2*c0);
    b2 = b0+4*c0*t2;
    tf = (b0+4*c0*t2 - vf)/(2*c0);
    a2 = a0 + b0*t2 + c0*t2^2 - b2*t2 - c2*t2^2;  
    if(t2>tf)||(t2<0)
        t2 = (-b0 - m)/(2*c0);
        b2 = b0+4*c0*t2;
        tf = (b0+4*c0*t2 - vf)/(2*c0);
        a2 = a0 + b0*t2 + c0*t2^2 - b2*t2 - c2*t2^2; 
    end

else %LSPB bool = 1, linear segment is needed
    b1 = n*vMax;
    t1 = (n*vMax - b0)/(2*c0);
    a1 = a0 + b0*t1 + c0*t1^2 - b1*t1;
    t2 = (xf - a1 + (n^2*vMax^2)/(4*c2) - (vf^2)/(4*c2))/b1;
    tf = (2*c2*t2 + vf - n*vMax)/(2*c2);
    b2 = n*vMax - 2*c2*t2;
    a2 = xf - b2*tf - c2*tf^2;
    
end

end

== matlab function pjh_pid/MJ_V_compen ==
  data: q input size=[1 6]; C_tau output size=[1 6]; qd input size=[1 6]
function C_tau = MJ_C_vector_pack( q, qd)
    C_tau  = MJ_C_vector( q, qd);
end
